simulink model "w1p4"  (R2020b)
settings: Solver=VariableStepAuto  StartTime=0.0  StopTime=10.0  RelTol=1e-3
settings Model: Creator=WELCOME  LastModifiedBy=WELCOME

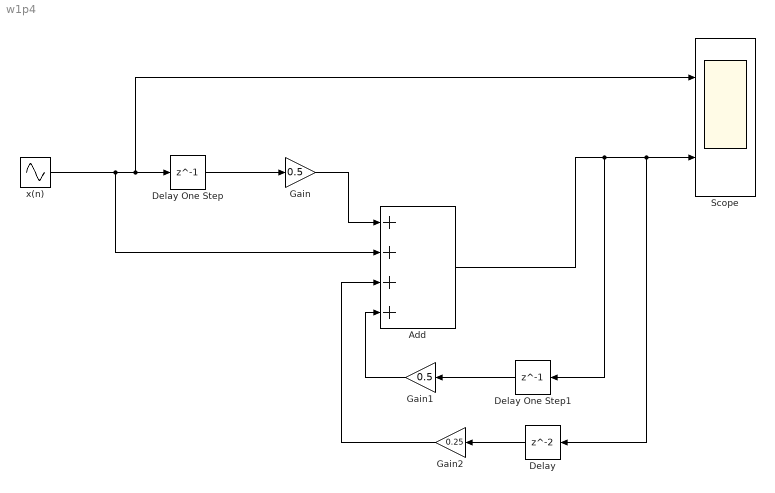
== system w1p4 ==
  Add : Sum  Inputs=++++
  Delay : Delay
  Delay One Step : Delay  DelayLength=1
  Delay One Step1 : Delay  DelayLength=1
  Gain : Gain  Gain=0.5
  Gain1 : Gain  Gain=0.5
  Gain2 : Gain  Gain=0.25
  Scope : Scope  NumInputPorts=2
  x(n) : Sin  SampleTime=0
  wires:
  x(n)/1 -> Add/2, Scope/1, Delay One Step/1
  Delay One Step/1 -> Gain/1
  Gain/1 -> Add/1
  Gain1/1 -> Add/4
  Gain2/1 -> Add/3
  Delay One Step1/1 -> Gain1/1
  Delay/1 -> Gain2/1
  Add/1 -> Delay One Step1/1, Delay/1, Scope/2
